simulink model "StepperMotorMusicPulseOutput2"  (R2019b)
settings: Solver=FixedStepDiscrete  StartTime=0.0  StopTime=10.0  FixedStep=T_s  RelTol=1e-3  EnableMultiTasking=on
undefined symbols (not defined in the file): DiscIntNeverNeededParam, SYM_nu, T_s, t_sim
libraries: dspsigops x36, sbox2 x3
settings Model: Creator=haketa  LastModifiedBy=STEPPERMOTOR
settings DataIOCC: LimitDataPoints=on  SaveFormat=Array  SignalLoggingSaveFormat=ModelDataLogs  ReturnWorkspaceOutputs=off
settings OptimizationCC: BlockReduction=off  OptimizeBlockIOStorage=off  BufferReuse=off  GlobalBufferReuse=off  ExpressionFolding=off  ExpressionDepthLimit=2147483647  LocalBlockOutputs=off  InitFltsAndDblsToZero=on  LifeSpan=inf  OptimizeDataStoreBuffers=off  BusAssignmentInplaceUpdate=off
settings DebuggingCC: SaveWithParameterizedLinksMsg=none  UnderspecifiedInitializationDetection=Classic  MergeDetectMultiDrivingBlocksExec=none  SignalResolutionControl=TryResolveAllWithWarning  SolverPrmCheckMsg=warning  InheritedTsInSrcMsg=none  MultiTaskDSMMsg=warning  MultiTaskCondExecSysMsg=none  FcnCallInpInsideContextMsg=warning  StateNameClashWarn=warning  SFUnexpectedBacktrackingDiag=warning  SFNoUnconditionalDefaultTransitionDiag=warning  SFExecutionAtInitializationDiag=none  ArithmeticOperatorsInVariantConditions=warning
settings HardwareCC: ProdBitPerPointer=32  ProdBitPerSizeT=32  ProdBitPerPtrDiffT=32  ProdLargestAtomicFloat=None  ProdIntDivRoundTo=Undefined  ProdEndianess=Unspecified  ProdWordSize=32  ProdHWDeviceType=32-bit Generic
settings ModelReferenceCC: PropagateSignalLabelsOutOfModel=off
settings SFSimCC: SimUseLocalCustomCode=off  CustomCodeUndefinedFunction=UseInterfaceOnly
settings RTWCC: Description=MTT sBOXII Real-Time Target.  SystemTargetFile=sbox2.tlc  TemplateMakefile=sbox2.tmf  RTWUseLocalCustomCode=off  RTWCompilerOptimization=on
settings CodeAppCC: StateflowObjectComments=on
settings GRTTargetCC: TargetLangStandard=C89/C90 (ANSI)  MatFileLogging=off  UseToolchainInfoCompliant=off  RTWCAPISignals=on  RTWCAPIParams=on
settings ConfigComp: CovMetricSettings=dw  CovSaveCumulativeToWorkspaceVar=on  CovSaveSingleToWorkspaceVar=on  CovExternalEMLEnable=off  CovSFcnEnable=off

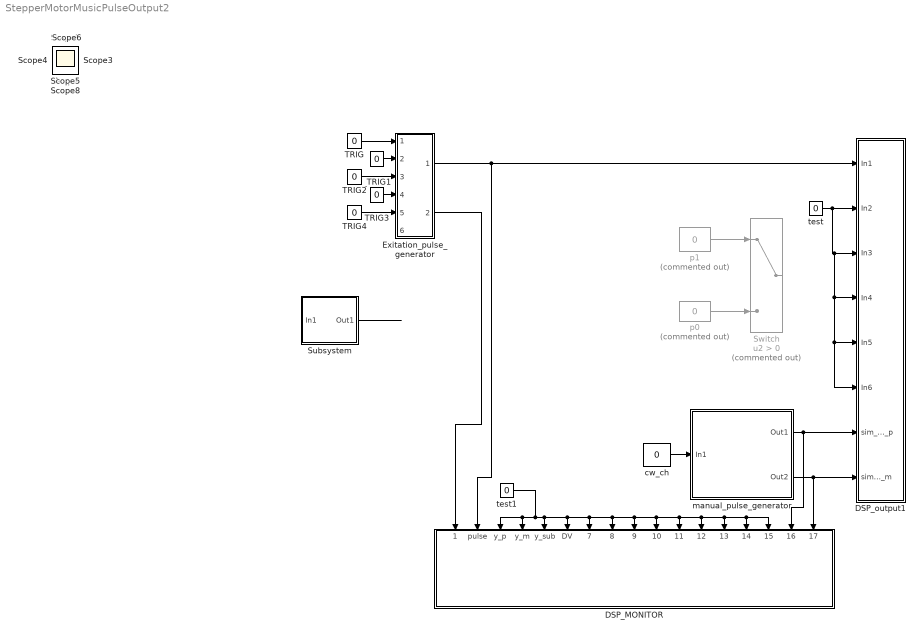
== system StepperMotorMusicPulseOutput2 ==
  DSP_MONITOR : Subsystem
  DSP_output1 : Subsystem
  Exitation_pulse_generator : Subsystem
  Subsystem : Subsystem
  Switch : Switch  Commented=on  Criteria=u2 > Threshold
  TRIG{,2..4} (4 alike) : Constant  Value=0  SampleTime=-1
  _TRIG1 : Constant  Value=0  SampleTime=-1
  cw_ch : Constant  Value=0  SampleTime=-1
  manual_pulse_generator : Subsystem
  p0 : Constant  Commented=on  Value=0  SampleTime=-1
  p1 : Constant  Commented=on  Value=0  SampleTime=-1
  test : Constant  Value=0  SampleTime=-1
  test1 : Constant  Value=0  SampleTime=-1
  Scope{,1..6,8} (8 alike) : Scope
  wires:
  TRIG4/1 -> Exitation_pulse_generator/5(In5)
  manual_pulse_generator/1(Out1) -> DSP_output1/7(sim_CW_p), DSP_MONITOR/16(hoge1)
  manual_pulse_generator/2(Out2) -> DSP_output1/8(sim_CW_m), DSP_MONITOR/17(hoge2)
  TRIG3/1 -> Exitation_pulse_generator/4(In4)
  p0/1 -> Switch/3
  _TRIG1/1 -> Exitation_pulse_generator/2(In2)
  TRIG/1 -> Exitation_pulse_generator/1(TRIG)
  Exitation_pulse_generator/1(sim_CW) -> DSP_output1/1(In1), DSP_MONITOR/2(pulse)
  TRIG2/1 -> Exitation_pulse_generator/3(In3)
  Exitation_pulse_generator/2(TRIG_parameter) -> DSP_MONITOR/1(DSP_SAVE_TRIG)
  test/1 -> DSP_output1/2(In2), DSP_output1/3(In3), DSP_output1/4(In4), DSP_output1/5(In5), DSP_output1/6(In6)
  ? -> Switch/2
  test1/1 -> DSP_MONITOR/4(y_m), DSP_MONITOR/3(y_p), DSP_MONITOR/15(CW_sim_sub), DSP_MONITOR/14(CW_sim_m), DSP_MONITOR/13(CW_sim_p), DSP_MONITOR/12(CW_mel_sub), DSP_MONITOR/11(CW_mel_m), DSP_MONITOR/10(CW_mel_p), DSP_MONITOR/9(u_analog), DSP_MONITOR/8(u_digital_sat), DSP_MONITOR/7(u_digital), DSP_MONITOR/6(DV), DSP_MONITOR/5(y_sub)
  p1/1 -> Switch/1
  cw_ch/1 -> manual_pulse_generator/1(In1)
  ? -> Subsystem/1(In1)
  Subsystem/1(Out1) -> ?

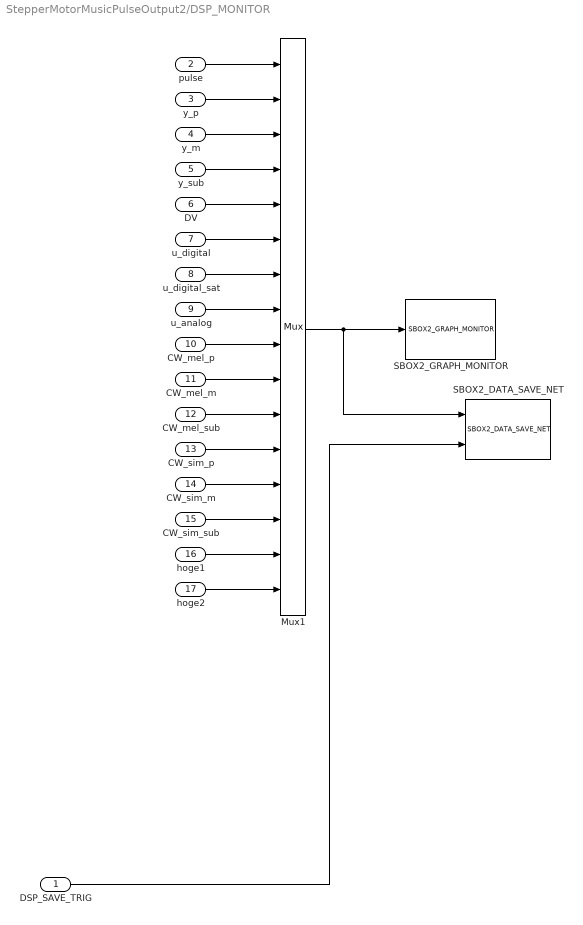
== system StepperMotorMusicPulseOutput2/DSP_MONITOR ==
  DSP_SAVE_TRIG : Inport
  pulse : Inport  Port=2
  y_p : Inport  Port=3
  y_m : Inport  Port=4
  y_sub : Inport  Port=5
  DV : Inport  Port=6
  u_digital : Inport  Port=7
  u_digital_sat : Inport  Port=8
  u_analog : Inport  Port=9
  CW_mel_p : Inport  Port=10
  CW_mel_m : Inport  Port=11
  CW_mel_sub : Inport  Port=12
  CW_sim_p : Inport  Port=13
  CW_sim_m : Inport  Port=14
  CW_sim_sub : Inport  Port=15
  hoge1 : Inport  Port=16
  hoge2 : Inport  Port=17
  Mux1 : Mux  Inputs=16
  SBOX2_DATA_SAVE_NET : sbox2/Network Data Save Devices/SBOX2_DATA_SAVE_NET  save_mode=ホストアプリケーション指示によるトリガ待ち  data_length=(t_sim/T_s)  pre_triger=0  sampletime=-1
  SBOX2_GRAPH_MONITOR : sbox2/Network Data Save Devices/SBOX2_GRAPH_MONITOR  sampletime=-1
  wires:
  DSP_SAVE_TRIG/1 -> SBOX2_DATA_SAVE_NET/2
  y_p/1 -> Mux1/2
  Mux1/1 -> SBOX2_DATA_SAVE_NET/1, SBOX2_GRAPH_MONITOR/1
  pulse/1 -> Mux1/1
  y_sub/1 -> Mux1/4
  u_digital/1 -> Mux1/6
  u_analog/1 -> Mux1/8
  u_digital_sat/1 -> Mux1/7
  DV/1 -> Mux1/5
  y_m/1 -> Mux1/3
  CW_mel_p/1 -> Mux1/9
  CW_mel_m/1 -> Mux1/10
  CW_mel_sub/1 -> Mux1/11
  CW_sim_p/1 -> Mux1/12
  CW_sim_m/1 -> Mux1/13
  CW_sim_sub/1 -> Mux1/14
  hoge1/1 -> Mux1/15
  hoge2/1 -> Mux1/16

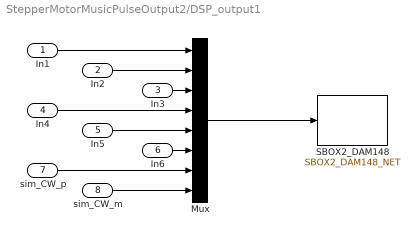
== system StepperMotorMusicPulseOutput2/DSP_output1 ==
  In1 : Inport
  In2 : Inport  Port=2
  In3 : Inport  Port=3
  In4 : Inport  Port=4
  In5 : Inport  Port=5
  In6 : Inport  Port=6
  sim_CW_p : Inport  Port=7
  sim_CW_m : Inport  Port=8
  Mux : Mux  Inputs=8
  SBOX2_DAM148 : sbox2/Analog I//O Devices/SBOX2_DAM148_NET  daStopCtrl1=0V出力  daStopCtrl2=0V出力  daStopCtrl3=0V出力  daStopCtrl4=0V出力  daStopCtrl5=0V出力  daStopCtrl6=0V出力  daStopCtrl7=0V出力  daStopCtrl8=0V出力  sampletime=-1
  wires:
  sim_CW_p/1 -> Mux/7
  Mux/1 -> SBOX2_DAM148/1
  In2/1 -> Mux/2
  In1/1 -> Mux/1
  In4/1 -> Mux/4
  In5/1 -> Mux/5
  In6/1 -> Mux/6
  sim_CW_m/1 -> Mux/8
  In3/1 -> Mux/3

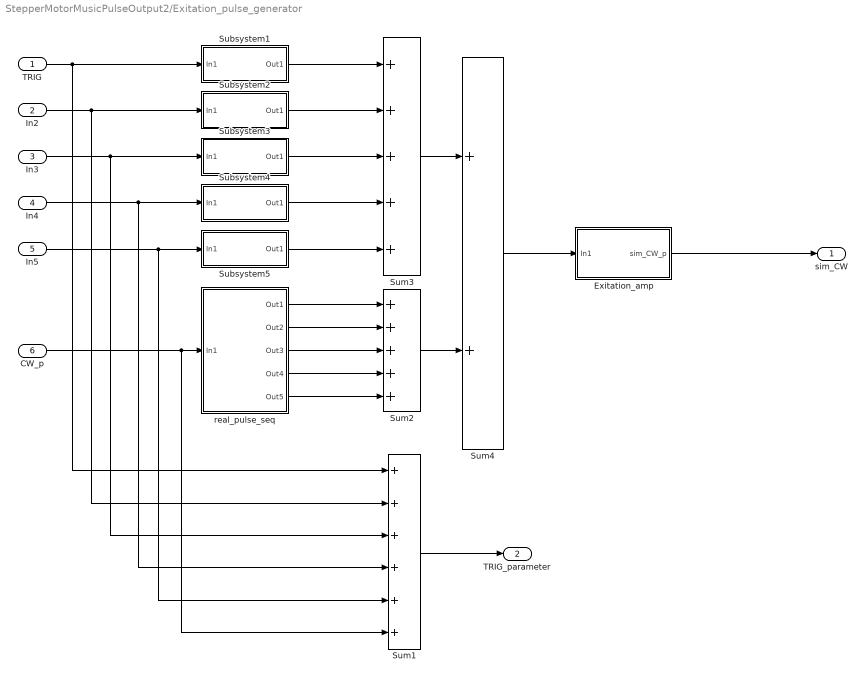
== system StepperMotorMusicPulseOutput2/Exitation_pulse_generator ==
  TRIG : Inport
  In2 : Inport  Port=2
  In3 : Inport  Port=3
  In4 : Inport  Port=4
  In5 : Inport  Port=5
  CW_p : Inport  Port=6
  Exitation_amp : Subsystem
  Subsystem1 : Subsystem
  Subsystem2 : Subsystem
  Subsystem3 : Subsystem
  Subsystem4 : Subsystem
  Subsystem5 : Subsystem
  Sum1 : Sum  Inputs=++++++
  Sum2 : Sum  Inputs=+++++
  Sum3 : Sum  Inputs=+++++
  Sum4 : Sum
  real_pulse_seq : Subsystem
  sim_CW : Outport
  TRIG_parameter : Outport  Port=2
  wires:
  Sum4/1 -> Exitation_amp/1(In1)
  Exitation_amp/1(sim_CW_p) -> sim_CW/1
  TRIG/1 -> Subsystem1/1(In1), Sum1/1
  Subsystem1/1(Out1) -> Sum3/1
  In2/1 -> Subsystem2/1(In1), Sum1/2
  In3/1 -> Subsystem3/1(In1), Sum1/3
  In4/1 -> Subsystem4/1(In1), Sum1/4
  In5/1 -> Subsystem5/1(In1), Sum1/5
  CW_p/1 -> Sum1/6, real_pulse_seq/1(In1)
  Subsystem2/1(Out1) -> Sum3/2
  Subsystem3/1(Out1) -> Sum3/3
  Subsystem4/1(Out1) -> Sum3/4
  Subsystem5/1(Out1) -> Sum3/5
  real_pulse_seq/1(Out1) -> Sum2/1
  real_pulse_seq/2(Out2) -> Sum2/2
  real_pulse_seq/3(Out3) -> Sum2/3
  real_pulse_seq/4(Out4) -> Sum2/4
  Sum1/1 -> TRIG_parameter/1
  real_pulse_seq/5(Out5) -> Sum2/5
  Sum2/1 -> Sum4/2
  Sum3/1 -> Sum4/1

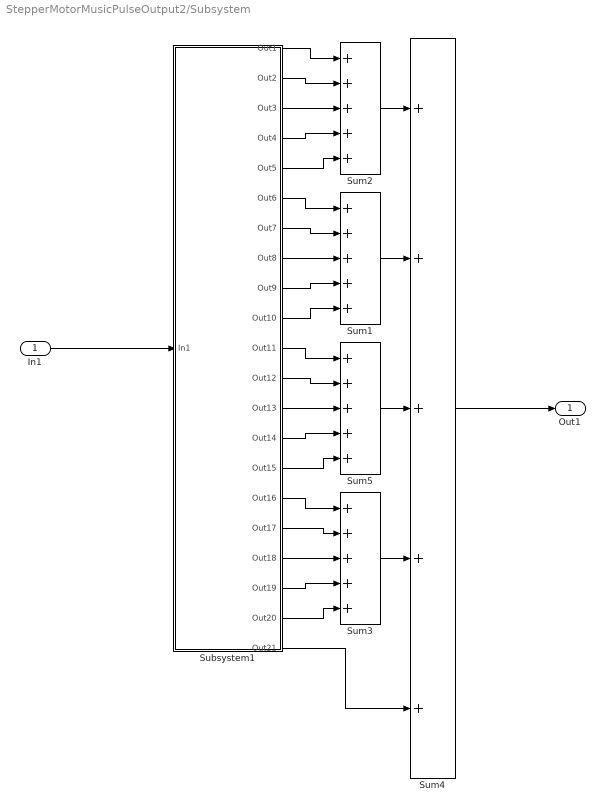
== system StepperMotorMusicPulseOutput2/Subsystem ==
  In1 : Inport
  Subsystem1 : Subsystem
  Sum{1..5} (5 alike) : Sum  Inputs=+++++
  Out1 : Outport
  wires:
  Subsystem1/17(Out17) -> Sum3/2
  Subsystem1/7(Out7) -> Sum1/2
  Subsystem1/1(Out1) -> Sum2/1
  Sum3/1 -> Sum4/4
  Subsystem1/20(Out20) -> Sum3/5
  Subsystem1/9(Out9) -> Sum1/4
  Subsystem1/4(Out4) -> Sum2/4
  Subsystem1/21(Out21) -> Sum4/5
  Subsystem1/18(Out18) -> Sum3/3
  Subsystem1/12(Out12) -> Sum5/2
  Sum2/1 -> Sum4/1
  Subsystem1/6(Out6) -> Sum1/1
  Subsystem1/5(Out5) -> Sum2/5
  Subsystem1/16(Out16) -> Sum3/1
  Subsystem1/15(Out15) -> Sum5/5
  Subsystem1/13(Out13) -> Sum5/3
  Sum5/1 -> Sum4/3
  Sum1/1 -> Sum4/2
  Subsystem1/8(Out8) -> Sum1/3
  Subsystem1/10(Out10) -> Sum1/5
  Subsystem1/3(Out3) -> Sum2/3
  Subsystem1/11(Out11) -> Sum5/1
  Subsystem1/14(Out14) -> Sum5/4
  Subsystem1/19(Out19) -> Sum3/4
  Subsystem1/2(Out2) -> Sum2/2
  Sum4/1 -> Out1/1
  In1/1 -> Subsystem1/1(In1)

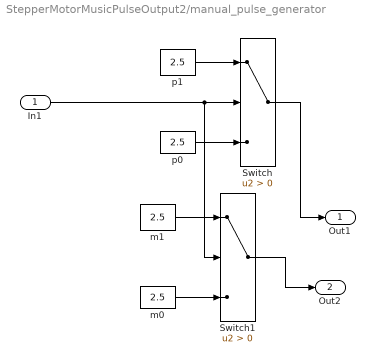
== system StepperMotorMusicPulseOutput2/manual_pulse_generator ==
  In1 : Inport
  Switch : Switch  Criteria=u2 > Threshold
  Switch1 : Switch  Criteria=u2 > Threshold
  m0 : Constant  Value=2.5  SampleTime=-1
  m1 : Constant  Value=2.5  SampleTime=-1
  p0 : Constant  Value=2.5  SampleTime=-1
  p1 : Constant  Value=2.5  SampleTime=-1
  Out1 : Outport
  Out2 : Outport  Port=2
  wires:
  Switch1/1 -> Out2/1
  In1/1 -> Switch1/2, Switch/2
  p1/1 -> Switch/1
  p0/1 -> Switch/3
  Switch/1 -> Out1/1
  m0/1 -> Switch1/3
  m1/1 -> Switch1/1

== system StepperMotorMusicPulseOutput2/Exitation_pulse_generator/Exitation_amp ==
  In1 : Inport
  Constant3 : Constant  Value=4.5  SampleTime=-1
  Gain5 : Gain  Gain=-1
  Switch : Switch  Criteria=u2 > Threshold
  sim_CW_p : Outport
  wires:
  Constant3/1 -> Switch/1, Gain5/1
  Gain5/1 -> Switch/3  "DV"
  Switch/1 -> sim_CW_p/1
  In1/1 -> Switch/2

== system StepperMotorMusicPulseOutput2/Exitation_pulse_generator/Subsystem1 ==
  In1 : Inport
  Constant3 : Constant  Value=0  SampleTime=-1
  Pulse Generator : DiscretePulseGenerator  PulseType=Time based  Period=T_s*2  PulseWidth=50
  Resettable Subsystem : Subsystem  TreatAsAtomicUnit=on
  Switch : Switch  Criteria=u2 > Threshold
  Out1 : Outport
  wires:
  In1/1 -> Switch/2, Resettable Subsystem/Reset
  Pulse Generator/1 -> Switch/1
  Constant3/1 -> Switch/3
  Resettable Subsystem/1(Out1) -> Out1/1
  Switch/1 -> Resettable Subsystem/1(In1)

== system StepperMotorMusicPulseOutput2/Exitation_pulse_generator/Subsystem2 ==
  In1 : Inport
  Constant3 : Constant  Value=0  SampleTime=-1
  Pulse Generator : DiscretePulseGenerator  PulseType=Time based  Period=T_s*2  PulseWidth=50
  Resettable Subsystem : Subsystem  TreatAsAtomicUnit=on
  Switch : Switch  Criteria=u2 > Threshold
  Out1 : Outport
  wires:
  Switch/1 -> Resettable Subsystem/1(In1)
  Resettable Subsystem/1(Out1) -> Out1/1
  Constant3/1 -> Switch/3
  Pulse Generator/1 -> Switch/1
  In1/1 -> Resettable Subsystem/Reset, Switch/2

== system StepperMotorMusicPulseOutput2/Exitation_pulse_generator/Subsystem3 ==
  In1 : Inport
  Constant3 : Constant  Value=0  SampleTime=-1
  Pulse Generator : DiscretePulseGenerator  PulseType=Time based  Period=T_s*2  PulseWidth=50
  Resettable Subsystem : Subsystem  TreatAsAtomicUnit=on
  Switch : Switch  Criteria=u2 > Threshold
  Out1 : Outport
  wires:
  In1/1 -> Switch/2, Resettable Subsystem/Reset
  Pulse Generator/1 -> Switch/1
  Constant3/1 -> Switch/3
  Resettable Subsystem/1(Out1) -> Out1/1
  Switch/1 -> Resettable Subsystem/1(In1)

== system StepperMotorMusicPulseOutput2/Exitation_pulse_generator/Subsystem4 ==
  In1 : Inport
  Constant3 : Constant  Value=0  SampleTime=-1
  Pulse Generator : DiscretePulseGenerator  PulseType=Time based  Period=T_s*2  PulseWidth=50
  Resettable Subsystem : Subsystem  TreatAsAtomicUnit=on
  Switch : Switch  Criteria=u2 > Threshold
  Out1 : Outport
  wires:
  Switch/1 -> Resettable Subsystem/1(In1)
  Resettable Subsystem/1(Out1) -> Out1/1
  Constant3/1 -> Switch/3
  Pulse Generator/1 -> Switch/1
  In1/1 -> Resettable Subsystem/Reset, Switch/2

== system StepperMotorMusicPulseOutput2/Exitation_pulse_generator/Subsystem5 ==
  In1 : Inport
  Constant3 : Constant  Value=0  SampleTime=-1
  Pulse Generator : DiscretePulseGenerator  PulseType=Time based  Period=T_s*2  PulseWidth=50
  Resettable Subsystem : Subsystem  TreatAsAtomicUnit=on
  Switch : Switch  Criteria=u2 > Threshold
  Out1 : Outport
  wires:
  In1/1 -> Switch/2, Resettable Subsystem/Reset
  Pulse Generator/1 -> Switch/1
  Constant3/1 -> Switch/3
  Resettable Subsystem/1(Out1) -> Out1/1
  Switch/1 -> Resettable Subsystem/1(In1)

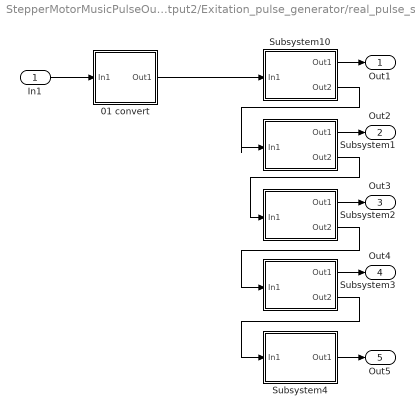
== system StepperMotorMusicPulseOutput2/Exitation_pulse_generator/real_pulse_seq ==
  In1 : Inport
  01 convert : Subsystem
  Subsystem1 : Subsystem
  Subsystem10 : Subsystem
  Subsystem2 : Subsystem
  Subsystem3 : Subsystem
  Subsystem4 : Subsystem
  Out1 : Outport
  Out2 : Outport  Port=2
  Out3 : Outport  Port=3
  Out4 : Outport  Port=4
  Out5 : Outport  Port=5
  wires:
  Subsystem2/1(Out1) -> Out3/1
  Subsystem1/1(Out1) -> Out2/1
  Subsystem10/1(Out1) -> Out1/1
  Subsystem1/2(Out2) -> Subsystem2/1(In1)
  Subsystem10/2(Out2) -> Subsystem1/1(In1)
  Subsystem2/2(Out2) -> Subsystem3/1(In1)
  Subsystem3/1(Out1) -> Out4/1
  In1/1 -> 01 convert/1(In1)
  01 convert/1(Out1) -> Subsystem10/1(In1)
  Subsystem3/2(Out2) -> Subsystem4/1(In1)
  Subsystem4/1(Out1) -> Out5/1

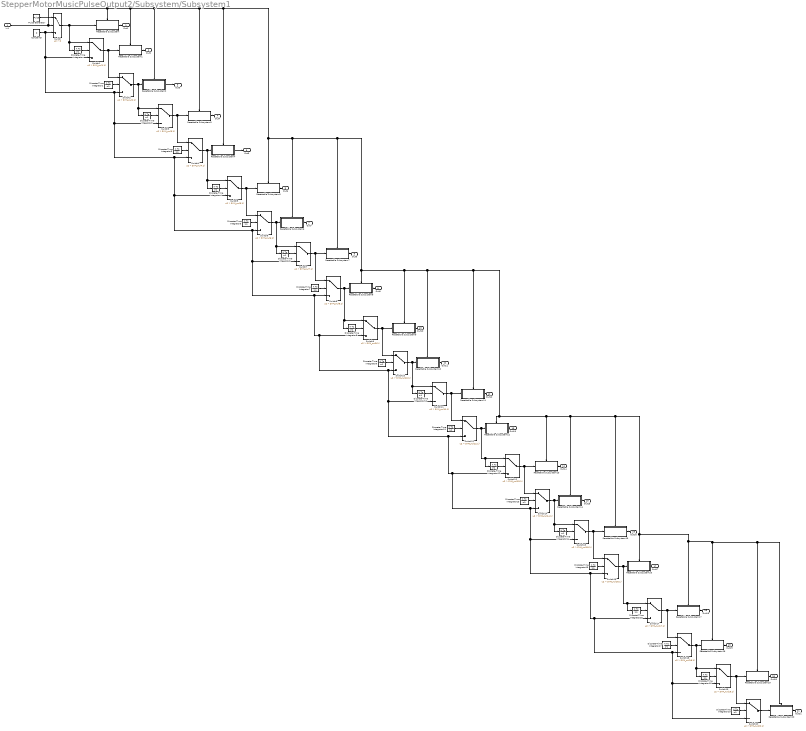
== system StepperMotorMusicPulseOutput2/Subsystem/Subsystem1 ==
  In1 : Inport
  Constant3 : Constant  Value=0  SampleTime=-1
  Discrete-Time Integrator{,1..19} (20 alike) : DiscreteIntegrator  SampleTime=-1  ICPrevOutput=DiscIntNeverNeededParam  ICPrevScaledInput=DiscIntNeverNeededParam
  Pulse Generator : DiscretePulseGenerator  PulseType=Time based  Period=T_s*2  PulseWidth=50
  Resettable Subsystem : Subsystem  TreatAsAtomicUnit=on
  Resettable Subsystem1 : Subsystem  TreatAsAtomicUnit=on
  Resettable Subsystem10 : Subsystem  TreatAsAtomicUnit=on
  Resettable Subsystem11 : Subsystem  TreatAsAtomicUnit=on
  Resettable Subsystem12 : Subsystem  TreatAsAtomicUnit=on
  Resettable Subsystem13 : Subsystem  TreatAsAtomicUnit=on
  Resettable Subsystem14 : Subsystem  TreatAsAtomicUnit=on
  Resettable Subsystem15 : Subsystem  TreatAsAtomicUnit=on
  Resettable Subsystem16 : Subsystem  TreatAsAtomicUnit=on
  Resettable Subsystem17 : Subsystem  TreatAsAtomicUnit=on
  Resettable Subsystem18 : Subsystem  TreatAsAtomicUnit=on
  Resettable Subsystem19 : Subsystem  TreatAsAtomicUnit=on
  Resettable Subsystem2 : Subsystem  TreatAsAtomicUnit=on
  Resettable Subsystem20 : Subsystem  TreatAsAtomicUnit=on
  Resettable Subsystem3 : Subsystem  TreatAsAtomicUnit=on
  Resettable Subsystem4 : Subsystem  TreatAsAtomicUnit=on
  Resettable Subsystem5 : Subsystem  TreatAsAtomicUnit=on
  Resettable Subsystem6 : Subsystem  TreatAsAtomicUnit=on
  Resettable Subsystem7 : Subsystem  TreatAsAtomicUnit=on
  Resettable Subsystem8 : Subsystem  TreatAsAtomicUnit=on
  Resettable Subsystem9 : Subsystem  TreatAsAtomicUnit=on
  Switch : Switch  Criteria=u2 > Threshold
  Switch1 : Switch  Criteria=u2 > Threshold  Threshold=SYM_nu(1,1)
  Switch10 : Switch  Criteria=u2 > Threshold  Threshold=SYM_nu(10,1)
  Switch11 : Switch  Criteria=u2 > Threshold  Threshold=SYM_nu(11,1)
  Switch12 : Switch  Criteria=u2 > Threshold  Threshold=SYM_nu(12,1)
  Switch13 : Switch  Criteria=u2 > Threshold  Threshold=SYM_nu(13,1)
  Switch14 : Switch  Criteria=u2 > Threshold  Threshold=SYM_nu(14,1)
  Switch15 : Switch  Criteria=u2 > Threshold  Threshold=SYM_nu(15,1)
  Switch16 : Switch  Criteria=u2 > Threshold  Threshold=SYM_nu(16,1)
  Switch17 : Switch  Criteria=u2 > Threshold  Threshold=SYM_nu(17,1)
  Switch18 : Switch  Criteria=u2 > Threshold  Threshold=SYM_nu(18,1)
  Switch19 : Switch  Criteria=u2 > Threshold  Threshold=SYM_nu(19,1)
  Switch2 : Switch  Criteria=u2 > Threshold  Threshold=SYM_nu(2,1)
  Switch20 : Switch  Criteria=u2 > Threshold  Threshold=SYM_nu(20,1)
  Switch3 : Switch  Criteria=u2 > Threshold  Threshold=SYM_nu(3,1)
  Switch4 : Switch  Criteria=u2 > Threshold  Threshold=SYM_nu(4,1)
  Switch5 : Switch  Criteria=u2 > Threshold  Threshold=SYM_nu(5,1)
  Switch6 : Switch  Criteria=u2 > Threshold  Threshold=SYM_nu(6,1)
  Switch7 : Switch  Criteria=u2 > Threshold  Threshold=SYM_nu(7,1)
  Switch8 : Switch  Criteria=u2 > Threshold  Threshold=SYM_nu(8,1)
  Switch9 : Switch  Criteria=u2 > Threshold  Threshold=SYM_nu(9,1)
  Out1 : Outport
  Out2 : Outport  Port=2
  Out3 : Outport  Port=3
  Out4 : Outport  Port=4
  Out5 : Outport  Port=5
  Out6 : Outport  Port=6
  Out7 : Outport  Port=7
  Out8 : Outport  Port=8
  Out9 : Outport  Port=9
  Out10 : Outport  Port=10
  Out11 : Outport  Port=11
  Out12 : Outport  Port=12
  Out13 : Outport  Port=13
  Out14 : Outport  Port=14
  Out15 : Outport  Port=15
  Out16 : Outport  Port=16
  Out17 : Outport  Port=17
  Out18 : Outport  Port=18
  Out19 : Outport  Port=19
  Out20 : Outport  Port=20
  Out21 : Outport  Port=21
  wires:
  Pulse Generator/1 -> Switch/1
  Resettable Subsystem/1(Out1) -> Out1/1
  Switch/1 -> Discrete-Time Integrator/1, Switch1/1, Resettable Subsystem/1(In1)
  Discrete-Time Integrator/1 -> Switch1/2
  Discrete-Time Integrator1/1 -> Switch2/2
  Switch1/1 -> Switch2/1, Resettable Subsystem1/1(In1)
  Switch3/1 -> Resettable Subsystem3/1(In1), Switch4/1
  Discrete-Time Integrator3/1 -> Switch4/2
  Discrete-Time Integrator2/1 -> Switch3/2
  Switch2/1 -> Switch3/1, Discrete-Time Integrator2/1, Resettable Subsystem2/1(In1)
  Switch6/1 -> Resettable Subsystem6/1(In1), Discrete-Time Integrator6/1, Switch7/1
  Discrete-Time Integrator6/1 -> Switch7/2
  Discrete-Time Integrator7/1 -> Switch8/2
  Switch7/1 -> Switch8/1, Resettable Subsystem7/1(In1)
  Switch5/1 -> Resettable Subsystem5/1(In1), Switch6/1
  Discrete-Time Integrator5/1 -> Switch6/2
  Discrete-Time Integrator4/1 -> Switch5/2
  Switch4/1 -> Switch5/1, Discrete-Time Integrator4/1, Resettable Subsystem4/1(In1)
  Switch12/1 -> Resettable Subsystem12/1(In1), Discrete-Time Integrator12/1, Switch13/1
  Discrete-Time Integrator12/1 -> Switch13/2
  Discrete-Time Integrator13/1 -> Switch14/2
  Switch13/1 -> Switch14/1, Resettable Subsystem13/1(In1)
  Switch15/1 -> Resettable Subsystem15/1(In1), Switch16/1
  Discrete-Time Integrator15/1 -> Switch16/2
  Discrete-Time Integrator14/1 -> Switch15/2
  Switch14/1 -> Switch15/1, Discrete-Time Integrator14/1, Resettable Subsystem14/1(In1)
  Switch10/1 -> Resettable Subsystem10/1(In1), Discrete-Time Integrator10/1, Switch11/1
  Discrete-Time Integrator10/1 -> Switch11/2
  Discrete-Time Integrator11/1 -> Switch12/2
  Switch11/1 -> Switch12/1, Resettable Subsystem11/1(In1)
  Switch9/1 -> Resettable Subsystem9/1(In1), Switch10/1
  Discrete-Time Integrator9/1 -> Switch10/2
  Discrete-Time Integrator8/1 -> Switch9/2
  Switch8/1 -> Discrete-Time Integrator8/1, Switch9/1, Resettable Subsystem8/1(In1)
  In1/1 -> Switch/2, Resettable Subsystem1/Reset, Resettable Subsystem2/Reset, Resettable Subsystem3/Reset, Resettable Subsystem7/Reset, Resettable Subsystem12/Reset, Resettable Subsystem13/Reset, Resettable Subsystem14/Reset, Resettable Subsystem19/Reset, Resettable Subsystem20/Reset, Resettable Subsystem18/Reset, Resettable Subsystem17/Reset, Resettable Subsystem16/Reset, Resettable Subsystem15/Reset, Resettable Subsystem11/Reset, Resettable Subsystem10/Reset, Resettable Subsystem9/Reset, Resettable Subsystem8/Reset, Resettable Subsystem6/Reset, Resettable Subsystem5/Reset, Resettable Subsystem4/Reset, Resettable Subsystem/Reset
  Discrete-Time Integrator19/1 -> Switch20/2
  Discrete-Time Integrator18/1 -> Switch19/2
  Switch18/1 -> Switch19/1, Discrete-Time Integrator18/1, Resettable Subsystem18/1(In1)
  Constant3/1 -> Switch3/3, Switch5/3, Switch6/3, Switch9/3, Switch10/3, Switch12/3, Switch15/3, Switch19/3, Switch20/3, Switch18/3, Switch17/3, Switch16/3, Switch14/3, Switch13/3, Switch11/3, Switch8/3, Switch7/3, Switch4/3, Switch2/3, Switch1/3, Switch/3
  Discrete-Time Integrator17/1 -> Switch18/2
  Discrete-Time Integrator16/1 -> Switch17/2
  Switch16/1 -> Discrete-Time Integrator16/1, Switch17/1, Resettable Subsystem16/1(In1)
  Switch20/1 -> Resettable Subsystem20/1(In1)
  Switch19/1 -> Resettable Subsystem19/1(In1), Switch20/1
  Switch17/1 -> Switch18/1, Resettable Subsystem17/1(In1)
  Resettable Subsystem1/1(Out1) -> Out2/1
  Resettable Subsystem2/1(Out1) -> Out3/1
  Resettable Subsystem3/1(Out1) -> Out4/1
  Resettable Subsystem4/1(Out1) -> Out5/1
  Resettable Subsystem5/1(Out1) -> Out6/1
  Resettable Subsystem6/1(Out1) -> Out7/1
  Resettable Subsystem7/1(Out1) -> Out8/1
  Resettable Subsystem8/1(Out1) -> Out9/1
  Resettable Subsystem9/1(Out1) -> Out10/1
  Resettable Subsystem10/1(Out1) -> Out11/1
  Resettable Subsystem11/1(Out1) -> Out12/1
  Resettable Subsystem12/1(Out1) -> Out13/1
  Resettable Subsystem13/1(Out1) -> Out14/1
  Resettable Subsystem14/1(Out1) -> Out15/1
  Resettable Subsystem15/1(Out1) -> Out16/1
  Resettable Subsystem16/1(Out1) -> Out17/1
  Resettable Subsystem17/1(Out1) -> Out18/1
  Resettable Subsystem18/1(Out1) -> Out19/1
  Resettable Subsystem19/1(Out1) -> Out20/1
  Resettable Subsystem20/1(Out1) -> Out21/1

== system StepperMotorMusicPulseOutput2/Exitation_pulse_generator/Subsystem1/Resettable Subsystem ==
  In1 : Inport
  Reset : ResetPort  DisableCoverage=on  ResetTriggerType=falling
  Triggered Signal From Workspace : dspsigops/Triggered Signal From Workspace  Signal=MusicPulse  TriggerType=Either edge  ic=0  SamplesPerFrame=1  OutputAfterFinalValue=Setting to zero  OutputFrames=off
      settings: SourceProductName=DSP System Toolbox  SourceProductBaseCode=DS
  Out1 : Outport
  wires:
  In1/1 -> Triggered Signal From Workspace/Trigger
  Triggered Signal From Workspace/1 -> Out1/1

== system StepperMotorMusicPulseOutput2/Exitation_pulse_generator/Subsystem2/Resettable Subsystem ==
  In1 : Inport
  Reset : ResetPort  DisableCoverage=on  ResetTriggerType=falling
  Triggered Signal From Workspace : dspsigops/Triggered Signal From Workspace  Signal=MusicPulse  TriggerType=Either edge  ic=0  SamplesPerFrame=1  OutputAfterFinalValue=Setting to zero  OutputFrames=off
      settings: SourceProductName=DSP System Toolbox  SourceProductBaseCode=DS
  Out1 : Outport
  wires:
  Triggered Signal From Workspace/1 -> Out1/1
  In1/1 -> Triggered Signal From Workspace/Trigger

== system StepperMotorMusicPulseOutput2/Exitation_pulse_generator/Subsystem3/Resettable Subsystem ==
  In1 : Inport
  Reset : ResetPort  DisableCoverage=on  ResetTriggerType=falling
  Triggered Signal From Workspace : dspsigops/Triggered Signal From Workspace  Signal=MusicPulse  TriggerType=Either edge  ic=0  SamplesPerFrame=1  OutputAfterFinalValue=Setting to zero  OutputFrames=off
      settings: SourceProductName=DSP System Toolbox  SourceProductBaseCode=DS
  Out1 : Outport
  wires:
  In1/1 -> Triggered Signal From Workspace/Trigger
  Triggered Signal From Workspace/1 -> Out1/1

== system StepperMotorMusicPulseOutput2/Exitation_pulse_generator/Subsystem4/Resettable Subsystem ==
  In1 : Inport
  Reset : ResetPort  DisableCoverage=on  ResetTriggerType=falling
  Triggered Signal From Workspace : dspsigops/Triggered Signal From Workspace  Signal=MusicPulse  TriggerType=Either edge  ic=0  SamplesPerFrame=1  OutputAfterFinalValue=Setting to zero  OutputFrames=off
      settings: SourceProductName=DSP System Toolbox  SourceProductBaseCode=DS
  Out1 : Outport
  wires:
  Triggered Signal From Workspace/1 -> Out1/1
  In1/1 -> Triggered Signal From Workspace/Trigger

== system StepperMotorMusicPulseOutput2/Exitation_pulse_generator/Subsystem5/Resettable Subsystem ==
  In1 : Inport
  Reset : ResetPort  DisableCoverage=on  ResetTriggerType=falling
  Triggered Signal From Workspace : dspsigops/Triggered Signal From Workspace  Signal=MusicPulse  TriggerType=Either edge  ic=0  SamplesPerFrame=1  OutputAfterFinalValue=Setting to zero  OutputFrames=off
      settings: SourceProductName=DSP System Toolbox  SourceProductBaseCode=DS
  Out1 : Outport
  wires:
  In1/1 -> Triggered Signal From Workspace/Trigger
  Triggered Signal From Workspace/1 -> Out1/1

== system StepperMotorMusicPulseOutput2/Exitation_pulse_generator/real_pulse_seq/01 convert ==
  In1 : Inport
  Constant1 : Constant  SampleTime=-1
  Constant3 : Constant  Value=0  SampleTime=-1
  Switch : Switch  Criteria=u2 > Threshold  Threshold=0.5
  Out1 : Outport
  wires:
  Constant3/1 -> Switch/3
  Switch/1 -> Out1/1
  Constant1/1 -> Switch/1
  In1/1 -> Switch/2

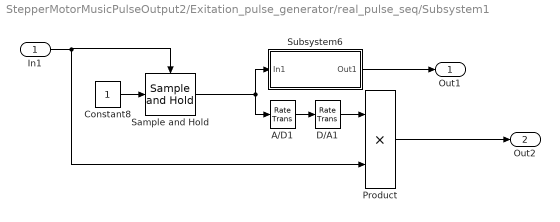
== system StepperMotorMusicPulseOutput2/Exitation_pulse_generator/real_pulse_seq/Subsystem1 ==
  In1 : Inport
  A/D1 : RateTransition  OutPortSampleTime=t_sim
  Constant8 : Constant  SampleTime=-1
  D/A1 : RateTransition  OutPortSampleTime=T_s
  Product : Product
  Sample and Hold : dspsigops/Sample and Hold  trig=Rising edge  initCond=0  latchinput=off
  Subsystem6 : Subsystem
  Out1 : Outport
  Out2 : Outport  Port=2
  wires:
  D/A1/1 -> Product/1
  A/D1/1 -> D/A1/1
  Sample and Hold/1 -> Subsystem6/1(In1), A/D1/1
  Subsystem6/1(Out1) -> Out1/1
  Product/1 -> Out2/1
  In1/1 -> Sample and Hold/Trigger, Product/2
  Constant8/1 -> Sample and Hold/1

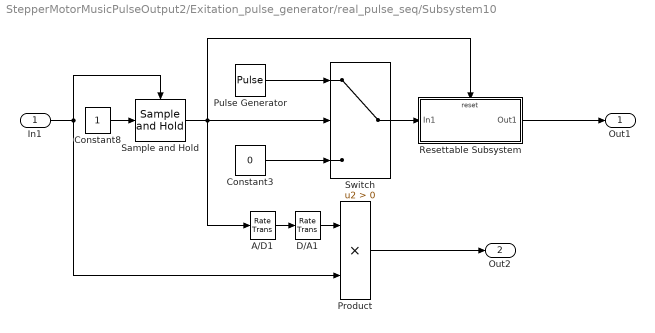
== system StepperMotorMusicPulseOutput2/Exitation_pulse_generator/real_pulse_seq/Subsystem10 ==
  In1 : Inport
  A/D1 : RateTransition  OutPortSampleTime=t_sim
  Constant3 : Constant  Value=0  SampleTime=-1
  Constant8 : Constant  SampleTime=-1
  D/A1 : RateTransition  OutPortSampleTime=T_s
  Product : Product
  Pulse Generator : DiscretePulseGenerator  PulseType=Time based  Period=T_s*2  PulseWidth=50
  Resettable Subsystem : Subsystem  TreatAsAtomicUnit=on
  Sample and Hold : dspsigops/Sample and Hold  trig=Rising edge  initCond=0  latchinput=off
  Switch : Switch  Criteria=u2 > Threshold
  Out1 : Outport
  Out2 : Outport  Port=2
  wires:
  Product/1 -> Out2/1
  Resettable Subsystem/1(Out1) -> Out1/1
  A/D1/1 -> D/A1/1
  D/A1/1 -> Product/1
  Constant8/1 -> Sample and Hold/1
  In1/1 -> Sample and Hold/Trigger, Product/2
  Sample and Hold/1 -> Switch/2, A/D1/1, Resettable Subsystem/Reset
  Pulse Generator/1 -> Switch/1
  Constant3/1 -> Switch/3
  Switch/1 -> Resettable Subsystem/1(In1)

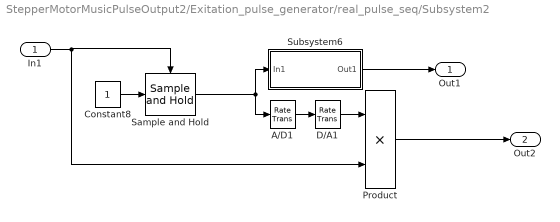
== system StepperMotorMusicPulseOutput2/Exitation_pulse_generator/real_pulse_seq/Subsystem2 ==
  In1 : Inport
  A/D1 : RateTransition  OutPortSampleTime=t_sim
  Constant8 : Constant  SampleTime=-1
  D/A1 : RateTransition  OutPortSampleTime=T_s
  Product : Product
  Sample and Hold : dspsigops/Sample and Hold  trig=Rising edge  initCond=0  latchinput=off
  Subsystem6 : Subsystem
  Out1 : Outport
  Out2 : Outport  Port=2
  wires:
  Constant8/1 -> Sample and Hold/1
  In1/1 -> Product/2, Sample and Hold/Trigger
  Product/1 -> Out2/1
  Subsystem6/1(Out1) -> Out1/1
  Sample and Hold/1 -> A/D1/1, Subsystem6/1(In1)
  A/D1/1 -> D/A1/1
  D/A1/1 -> Product/1

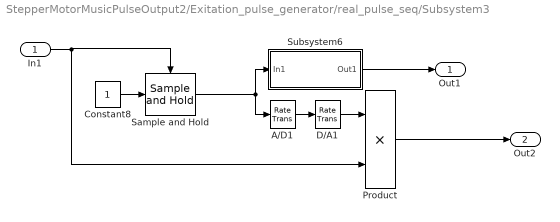
== system StepperMotorMusicPulseOutput2/Exitation_pulse_generator/real_pulse_seq/Subsystem3 ==
  In1 : Inport
  A/D1 : RateTransition  OutPortSampleTime=t_sim
  Constant8 : Constant  SampleTime=-1
  D/A1 : RateTransition  OutPortSampleTime=T_s
  Product : Product
  Sample and Hold : dspsigops/Sample and Hold  trig=Rising edge  initCond=0  latchinput=off
  Subsystem6 : Subsystem
  Out1 : Outport
  Out2 : Outport  Port=2
  wires:
  D/A1/1 -> Product/1
  A/D1/1 -> D/A1/1
  Sample and Hold/1 -> Subsystem6/1(In1), A/D1/1
  Subsystem6/1(Out1) -> Out1/1
  Product/1 -> Out2/1
  In1/1 -> Sample and Hold/Trigger, Product/2
  Constant8/1 -> Sample and Hold/1

== system StepperMotorMusicPulseOutput2/Exitation_pulse_generator/real_pulse_seq/Subsystem4 ==
  In1 : Inport
  Constant8 : Constant  SampleTime=-1
  Sample and Hold : dspsigops/Sample and Hold  trig=Rising edge  initCond=0  latchinput=off
  Subsystem6 : Subsystem
  Out1 : Outport
  wires:
  Constant8/1 -> Sample and Hold/1
  In1/1 -> Sample and Hold/Trigger
  Subsystem6/1(Out1) -> Out1/1
  Sample and Hold/1 -> Subsystem6/1(In1)

== system StepperMotorMusicPulseOutput2/Subsystem/Subsystem1/Resettable Subsystem ==
  In1 : Inport
  Reset : ResetPort  DisableCoverage=on  ResetTriggerType=falling
  Triggered Signal From Workspace : dspsigops/Triggered Signal From Workspace  Signal=MusicPulse01  TriggerType=Either edge  ic=0  SamplesPerFrame=1  OutputAfterFinalValue=Setting to zero  OutputFrames=off
      settings: SourceProductName=DSP System Toolbox  SourceProductBaseCode=DS
  Out1 : Outport
  wires:
  In1/1 -> Triggered Signal From Workspace/Trigger
  Triggered Signal From Workspace/1 -> Out1/1

== system StepperMotorMusicPulseOutput2/Subsystem/Subsystem1/Resettable Subsystem1 ==
  In1 : Inport
  Reset : ResetPort  DisableCoverage=on  ResetTriggerType=falling
  Triggered Signal From Workspace : dspsigops/Triggered Signal From Workspace  Signal=MusicPulse02  TriggerType=Either edge  ic=0  SamplesPerFrame=1  OutputAfterFinalValue=Setting to zero  OutputFrames=off
      settings: SourceProductName=DSP System Toolbox  SourceProductBaseCode=DS
  Out1 : Outport
  wires:
  Triggered Signal From Workspace/1 -> Out1/1
  In1/1 -> Triggered Signal From Workspace/Trigger

== system StepperMotorMusicPulseOutput2/Subsystem/Subsystem1/Resettable Subsystem10 ==
  In1 : Inport
  Reset : ResetPort  DisableCoverage=on  ResetTriggerType=falling
  Triggered Signal From Workspace : dspsigops/Triggered Signal From Workspace  Signal=MusicPulse11  TriggerType=Either edge  ic=0  SamplesPerFrame=1  OutputAfterFinalValue=Setting to zero  OutputFrames=off
      settings: SourceProductName=DSP System Toolbox  SourceProductBaseCode=DS
  Out1 : Outport
  wires:
  Triggered Signal From Workspace/1 -> Out1/1
  In1/1 -> Triggered Signal From Workspace/Trigger

== system StepperMotorMusicPulseOutput2/Subsystem/Subsystem1/Resettable Subsystem11 ==
  In1 : Inport
  Reset : ResetPort  DisableCoverage=on  ResetTriggerType=falling
  Triggered Signal From Workspace : dspsigops/Triggered Signal From Workspace  Signal=MusicPulse12  TriggerType=Either edge  ic=0  SamplesPerFrame=1  OutputAfterFinalValue=Setting to zero  OutputFrames=off
      settings: SourceProductName=DSP System Toolbox  SourceProductBaseCode=DS
  Out1 : Outport
  wires:
  Triggered Signal From Workspace/1 -> Out1/1
  In1/1 -> Triggered Signal From Workspace/Trigger

== system StepperMotorMusicPulseOutput2/Subsystem/Subsystem1/Resettable Subsystem12 ==
  In1 : Inport
  Reset : ResetPort  DisableCoverage=on  ResetTriggerType=falling
  Triggered Signal From Workspace : dspsigops/Triggered Signal From Workspace  Signal=MusicPulse13  TriggerType=Either edge  ic=0  SamplesPerFrame=1  OutputAfterFinalValue=Setting to zero  OutputFrames=off
      settings: SourceProductName=DSP System Toolbox  SourceProductBaseCode=DS
  Out1 : Outport
  wires:
  In1/1 -> Triggered Signal From Workspace/Trigger
  Triggered Signal From Workspace/1 -> Out1/1

== system StepperMotorMusicPulseOutput2/Subsystem/Subsystem1/Resettable Subsystem13 ==
  In1 : Inport
  Reset : ResetPort  DisableCoverage=on  ResetTriggerType=falling
  Triggered Signal From Workspace : dspsigops/Triggered Signal From Workspace  Signal=MusicPulse14  TriggerType=Either edge  ic=0  SamplesPerFrame=1  OutputAfterFinalValue=Setting to zero  OutputFrames=off
      settings: SourceProductName=DSP System Toolbox  SourceProductBaseCode=DS
  Out1 : Outport
  wires:
  Triggered Signal From Workspace/1 -> Out1/1
  In1/1 -> Triggered Signal From Workspace/Trigger

== system StepperMotorMusicPulseOutput2/Subsystem/Subsystem1/Resettable Subsystem14 ==
  In1 : Inport
  Reset : ResetPort  DisableCoverage=on  ResetTriggerType=falling
  Triggered Signal From Workspace : dspsigops/Triggered Signal From Workspace  Signal=MusicPulse15  TriggerType=Either edge  ic=0  SamplesPerFrame=1  OutputAfterFinalValue=Setting to zero  OutputFrames=off
      settings: SourceProductName=DSP System Toolbox  SourceProductBaseCode=DS
  Out1 : Outport
  wires:
  In1/1 -> Triggered Signal From Workspace/Trigger
  Triggered Signal From Workspace/1 -> Out1/1

== system StepperMotorMusicPulseOutput2/Subsystem/Subsystem1/Resettable Subsystem15 ==
  In1 : Inport
  Reset : ResetPort  DisableCoverage=on  ResetTriggerType=falling
  Triggered Signal From Workspace : dspsigops/Triggered Signal From Workspace  Signal=MusicPulse16  TriggerType=Either edge  ic=0  SamplesPerFrame=1  OutputAfterFinalValue=Setting to zero  OutputFrames=off
      settings: SourceProductName=DSP System Toolbox  SourceProductBaseCode=DS
  Out1 : Outport
  wires:
  In1/1 -> Triggered Signal From Workspace/Trigger
  Triggered Signal From Workspace/1 -> Out1/1

== system StepperMotorMusicPulseOutput2/Subsystem/Subsystem1/Resettable Subsystem16 ==
  In1 : Inport
  Reset : ResetPort  DisableCoverage=on  ResetTriggerType=falling
  Triggered Signal From Workspace : dspsigops/Triggered Signal From Workspace  Signal=MusicPulse17  TriggerType=Either edge  ic=0  SamplesPerFrame=1  OutputAfterFinalValue=Setting to zero  OutputFrames=off
      settings: SourceProductName=DSP System Toolbox  SourceProductBaseCode=DS
  Out1 : Outport
  wires:
  Triggered Signal From Workspace/1 -> Out1/1
  In1/1 -> Triggered Signal From Workspace/Trigger

== system StepperMotorMusicPulseOutput2/Subsystem/Subsystem1/Resettable Subsystem17 ==
  In1 : Inport
  Reset : ResetPort  DisableCoverage=on  ResetTriggerType=falling
  Triggered Signal From Workspace : dspsigops/Triggered Signal From Workspace  Signal=MusicPulse18  TriggerType=Either edge  ic=0  SamplesPerFrame=1  OutputAfterFinalValue=Setting to zero  OutputFrames=off
      settings: SourceProductName=DSP System Toolbox  SourceProductBaseCode=DS
  Out1 : Outport
  wires:
  Triggered Signal From Workspace/1 -> Out1/1
  In1/1 -> Triggered Signal From Workspace/Trigger

== system StepperMotorMusicPulseOutput2/Subsystem/Subsystem1/Resettable Subsystem18 ==
  In1 : Inport
  Reset : ResetPort  DisableCoverage=on  ResetTriggerType=falling
  Triggered Signal From Workspace : dspsigops/Triggered Signal From Workspace  Signal=MusicPulse19  TriggerType=Either edge  ic=0  SamplesPerFrame=1  OutputAfterFinalValue=Setting to zero  OutputFrames=off
      settings: SourceProductName=DSP System Toolbox  SourceProductBaseCode=DS
  Out1 : Outport
  wires:
  In1/1 -> Triggered Signal From Workspace/Trigger
  Triggered Signal From Workspace/1 -> Out1/1

== system StepperMotorMusicPulseOutput2/Subsystem/Subsystem1/Resettable Subsystem19 ==
  In1 : Inport
  Reset : ResetPort  DisableCoverage=on  ResetTriggerType=falling
  Triggered Signal From Workspace : dspsigops/Triggered Signal From Workspace  Signal=MusicPulse20  TriggerType=Either edge  ic=0  SamplesPerFrame=1  OutputAfterFinalValue=Setting to zero  OutputFrames=off
      settings: SourceProductName=DSP System Toolbox  SourceProductBaseCode=DS
  Out1 : Outport
  wires:
  In1/1 -> Triggered Signal From Workspace/Trigger
  Triggered Signal From Workspace/1 -> Out1/1

== system StepperMotorMusicPulseOutput2/Subsystem/Subsystem1/Resettable Subsystem2 ==
  In1 : Inport
  Reset : ResetPort  DisableCoverage=on  ResetTriggerType=falling
  Triggered Signal From Workspace : dspsigops/Triggered Signal From Workspace  Signal=MusicPulse03  TriggerType=Either edge  ic=0  SamplesPerFrame=1  OutputAfterFinalValue=Setting to zero  OutputFrames=off
      settings: SourceProductName=DSP System Toolbox  SourceProductBaseCode=DS
  Out1 : Outport
  wires:
  In1/1 -> Triggered Signal From Workspace/Trigger
  Triggered Signal From Workspace/1 -> Out1/1

== system StepperMotorMusicPulseOutput2/Subsystem/Subsystem1/Resettable Subsystem20 ==
  In1 : Inport
  Reset : ResetPort  DisableCoverage=on  ResetTriggerType=falling
  Triggered Signal From Workspace : dspsigops/Triggered Signal From Workspace  Signal=MusicPulse21  TriggerType=Either edge  ic=0  SamplesPerFrame=1  OutputAfterFinalValue=Setting to zero  OutputFrames=off
      settings: SourceProductName=DSP System Toolbox  SourceProductBaseCode=DS
  Out1 : Outport
  wires:
  Triggered Signal From Workspace/1 -> Out1/1
  In1/1 -> Triggered Signal From Workspace/Trigger

== system StepperMotorMusicPulseOutput2/Subsystem/Subsystem1/Resettable Subsystem3 ==
  In1 : Inport
  Reset : ResetPort  DisableCoverage=on  ResetTriggerType=falling
  Triggered Signal From Workspace : dspsigops/Triggered Signal From Workspace  Signal=MusicPulse04  TriggerType=Either edge  ic=0  SamplesPerFrame=1  OutputAfterFinalValue=Setting to zero  OutputFrames=off
      settings: SourceProductName=DSP System Toolbox  SourceProductBaseCode=DS
  Out1 : Outport
  wires:
  In1/1 -> Triggered Signal From Workspace/Trigger
  Triggered Signal From Workspace/1 -> Out1/1

== system StepperMotorMusicPulseOutput2/Subsystem/Subsystem1/Resettable Subsystem4 ==
  In1 : Inport
  Reset : ResetPort  DisableCoverage=on  ResetTriggerType=falling
  Triggered Signal From Workspace : dspsigops/Triggered Signal From Workspace  Signal=MusicPulse05  TriggerType=Either edge  ic=0  SamplesPerFrame=1  OutputAfterFinalValue=Setting to zero  OutputFrames=off
      settings: SourceProductName=DSP System Toolbox  SourceProductBaseCode=DS
  Out1 : Outport
  wires:
  Triggered Signal From Workspace/1 -> Out1/1
  In1/1 -> Triggered Signal From Workspace/Trigger

== system StepperMotorMusicPulseOutput2/Subsystem/Subsystem1/Resettable Subsystem5 ==
  In1 : Inport
  Reset : ResetPort  DisableCoverage=on  ResetTriggerType=falling
  Triggered Signal From Workspace : dspsigops/Triggered Signal From Workspace  Signal=MusicPulse06  TriggerType=Either edge  ic=0  SamplesPerFrame=1  OutputAfterFinalValue=Setting to zero  OutputFrames=off
      settings: SourceProductName=DSP System Toolbox  SourceProductBaseCode=DS
  Out1 : Outport
  wires:
  In1/1 -> Triggered Signal From Workspace/Trigger
  Triggered Signal From Workspace/1 -> Out1/1

== system StepperMotorMusicPulseOutput2/Subsystem/Subsystem1/Resettable Subsystem6 ==
  In1 : Inport
  Reset : ResetPort  DisableCoverage=on  ResetTriggerType=falling
  Triggered Signal From Workspace : dspsigops/Triggered Signal From Workspace  Signal=MusicPulse07  TriggerType=Either edge  ic=0  SamplesPerFrame=1  OutputAfterFinalValue=Setting to zero  OutputFrames=off
      settings: SourceProductName=DSP System Toolbox  SourceProductBaseCode=DS
  Out1 : Outport
  wires:
  Triggered Signal From Workspace/1 -> Out1/1
  In1/1 -> Triggered Signal From Workspace/Trigger

== system StepperMotorMusicPulseOutput2/Subsystem/Subsystem1/Resettable Subsystem7 ==
  In1 : Inport
  Reset : ResetPort  DisableCoverage=on  ResetTriggerType=falling
  Triggered Signal From Workspace : dspsigops/Triggered Signal From Workspace  Signal=MusicPulse08  TriggerType=Either edge  ic=0  SamplesPerFrame=1  OutputAfterFinalValue=Setting to zero  OutputFrames=off
      settings: SourceProductName=DSP System Toolbox  SourceProductBaseCode=DS
  Out1 : Outport
  wires:
  Triggered Signal From Workspace/1 -> Out1/1
  In1/1 -> Triggered Signal From Workspace/Trigger

== system StepperMotorMusicPulseOutput2/Subsystem/Subsystem1/Resettable Subsystem8 ==
  In1 : Inport
  Reset : ResetPort  DisableCoverage=on  ResetTriggerType=falling
  Triggered Signal From Workspace : dspsigops/Triggered Signal From Workspace  Signal=MusicPulse09  TriggerType=Either edge  ic=0  SamplesPerFrame=1  OutputAfterFinalValue=Setting to zero  OutputFrames=off
      settings: SourceProductName=DSP System Toolbox  SourceProductBaseCode=DS
  Out1 : Outport
  wires:
  In1/1 -> Triggered Signal From Workspace/Trigger
  Triggered Signal From Workspace/1 -> Out1/1

== system StepperMotorMusicPulseOutput2/Subsystem/Subsystem1/Resettable Subsystem9 ==
  In1 : Inport
  Reset : ResetPort  DisableCoverage=on  ResetTriggerType=falling
  Triggered Signal From Workspace : dspsigops/Triggered Signal From Workspace  Signal=MusicPulse10  TriggerType=Either edge  ic=0  SamplesPerFrame=1  OutputAfterFinalValue=Setting to zero  OutputFrames=off
      settings: SourceProductName=DSP System Toolbox  SourceProductBaseCode=DS
  Out1 : Outport
  wires:
  In1/1 -> Triggered Signal From Workspace/Trigger
  Triggered Signal From Workspace/1 -> Out1/1

== system StepperMotorMusicPulseOutput2/Exitation_pulse_generator/real_pulse_seq/Subsystem1/Subsystem6 ==
  In1 : Inport
  Constant3 : Constant  Value=0  SampleTime=-1
  Pulse Generator : DiscretePulseGenerator  PulseType=Time based  Period=T_s*2  PulseWidth=50
  Resettable Subsystem : Subsystem  TreatAsAtomicUnit=on
  Switch : Switch  Criteria=u2 > Threshold
  Out1 : Outport
  wires:
  In1/1 -> Switch/2, Resettable Subsystem/Reset
  Pulse Generator/1 -> Switch/1
  Constant3/1 -> Switch/3
  Resettable Subsystem/1(Out1) -> Out1/1
  Switch/1 -> Resettable Subsystem/1(In1)

== system StepperMotorMusicPulseOutput2/Exitation_pulse_generator/real_pulse_seq/Subsystem10/Resettable Subsystem ==
  In1 : Inport
  Reset : ResetPort  DisableCoverage=on  ResetTriggerType=falling
  Triggered Signal From Workspace : dspsigops/Triggered Signal From Workspace  Signal=MusicPulse  TriggerType=Either edge  ic=0  SamplesPerFrame=1  OutputAfterFinalValue=Setting to zero  OutputFrames=off
      settings: SourceProductName=DSP System Toolbox  SourceProductBaseCode=DS
  Out1 : Outport
  wires:
  Triggered Signal From Workspace/1 -> Out1/1
  In1/1 -> Triggered Signal From Workspace/Trigger

== system StepperMotorMusicPulseOutput2/Exitation_pulse_generator/real_pulse_seq/Subsystem2/Subsystem6 ==
  In1 : Inport
  Constant3 : Constant  Value=0  SampleTime=-1
  Pulse Generator : DiscretePulseGenerator  PulseType=Time based  Period=T_s*2  PulseWidth=50
  Resettable Subsystem : Subsystem  TreatAsAtomicUnit=on
  Switch : Switch  Criteria=u2 > Threshold
  Out1 : Outport
  wires:
  Switch/1 -> Resettable Subsystem/1(In1)
  Resettable Subsystem/1(Out1) -> Out1/1
  Constant3/1 -> Switch/3
  Pulse Generator/1 -> Switch/1
  In1/1 -> Resettable Subsystem/Reset, Switch/2

== system StepperMotorMusicPulseOutput2/Exitation_pulse_generator/real_pulse_seq/Subsystem3/Subsystem6 ==
  In1 : Inport
  Constant3 : Constant  Value=0  SampleTime=-1
  Pulse Generator : DiscretePulseGenerator  PulseType=Time based  Period=T_s*2  PulseWidth=50
  Resettable Subsystem : Subsystem  TreatAsAtomicUnit=on
  Switch : Switch  Criteria=u2 > Threshold
  Out1 : Outport
  wires:
  In1/1 -> Switch/2, Resettable Subsystem/Reset
  Pulse Generator/1 -> Switch/1
  Constant3/1 -> Switch/3
  Resettable Subsystem/1(Out1) -> Out1/1
  Switch/1 -> Resettable Subsystem/1(In1)

== system StepperMotorMusicPulseOutput2/Exitation_pulse_generator/real_pulse_seq/Subsystem4/Subsystem6 ==
  In1 : Inport
  Constant3 : Constant  Value=0  SampleTime=-1
  Pulse Generator : DiscretePulseGenerator  PulseType=Time based  Period=T_s*2  PulseWidth=50
  Resettable Subsystem : Subsystem  TreatAsAtomicUnit=on
  Switch : Switch  Criteria=u2 > Threshold
  Out1 : Outport
  wires:
  Switch/1 -> Resettable Subsystem/1(In1)
  Resettable Subsystem/1(Out1) -> Out1/1
  Constant3/1 -> Switch/3
  Pulse Generator/1 -> Switch/1
  In1/1 -> Resettable Subsystem/Reset, Switch/2

== system StepperMotorMusicPulseOutput2/Exitation_pulse_generator/real_pulse_seq/Subsystem1/Subsystem6/Resettable Subsystem ==
  In1 : Inport
  Reset : ResetPort  DisableCoverage=on  ResetTriggerType=falling
  Triggered Signal From Workspace : dspsigops/Triggered Signal From Workspace  Signal=MusicPulse  TriggerType=Either edge  ic=0  SamplesPerFrame=1  OutputAfterFinalValue=Setting to zero  OutputFrames=off
      settings: SourceProductName=DSP System Toolbox  SourceProductBaseCode=DS
  Out1 : Outport
  wires:
  In1/1 -> Triggered Signal From Workspace/Trigger
  Triggered Signal From Workspace/1 -> Out1/1

== system StepperMotorMusicPulseOutput2/Exitation_pulse_generator/real_pulse_seq/Subsystem2/Subsystem6/Resettable Subsystem ==
  In1 : Inport
  Reset : ResetPort  DisableCoverage=on  ResetTriggerType=falling
  Triggered Signal From Workspace : dspsigops/Triggered Signal From Workspace  Signal=MusicPulse  TriggerType=Either edge  ic=0  SamplesPerFrame=1  OutputAfterFinalValue=Setting to zero  OutputFrames=off
      settings: SourceProductName=DSP System Toolbox  SourceProductBaseCode=DS
  Out1 : Outport
  wires:
  Triggered Signal From Workspace/1 -> Out1/1
  In1/1 -> Triggered Signal From Workspace/Trigger

== system StepperMotorMusicPulseOutput2/Exitation_pulse_generator/real_pulse_seq/Subsystem3/Subsystem6/Resettable Subsystem ==
  In1 : Inport
  Reset : ResetPort  DisableCoverage=on  ResetTriggerType=falling
  Triggered Signal From Workspace : dspsigops/Triggered Signal From Workspace  Signal=MusicPulse  TriggerType=Either edge  ic=0  SamplesPerFrame=1  OutputAfterFinalValue=Setting to zero  OutputFrames=off
      settings: SourceProductName=DSP System Toolbox  SourceProductBaseCode=DS
  Out1 : Outport
  wires:
  In1/1 -> Triggered Signal From Workspace/Trigger
  Triggered Signal From Workspace/1 -> Out1/1

== system StepperMotorMusicPulseOutput2/Exitation_pulse_generator/real_pulse_seq/Subsystem4/Subsystem6/Resettable Subsystem ==
  In1 : Inport
  Reset : ResetPort  DisableCoverage=on  ResetTriggerType=falling
  Triggered Signal From Workspace : dspsigops/Triggered Signal From Workspace  Signal=MusicPulse  TriggerType=Either edge  ic=0  SamplesPerFrame=1  OutputAfterFinalValue=Setting to zero  OutputFrames=off
      settings: SourceProductName=DSP System Toolbox  SourceProductBaseCode=DS
  Out1 : Outport
  wires:
  Triggered Signal From Workspace/1 -> Out1/1
  In1/1 -> Triggered Signal From Workspace/Trigger
